simulink model "t2_5_1"  (R2017b)
settings: Solver=VariableStepAuto  StartTime=0.0  StopTime=10.0  RelTol=1e-3
settings Model: Creator=zxy19  LastModifiedBy=zxy19

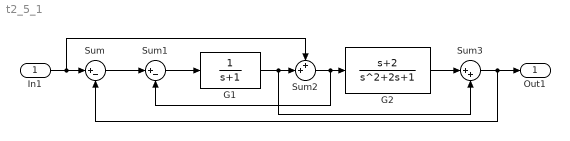
== system t2_5_1 ==
  In1 : Inport
  G1 : TransferFcn  Denominator=[1 1]  ContinuousStateAttributes='G1'
  G2 : TransferFcn  Numerator=[1 2]
  Sum : Sum  Inputs=|+-
  Sum1 : Sum  Inputs=|+-
  Sum2 : Sum  Inputs=++|
  Sum3 : Sum  Inputs=|++
  Out1 : Outport
  wires:
  Sum2/1 -> Sum1/2, G2/1
  G2/1 -> Sum3/1
  Sum3/1 -> Sum/2, Out1/1
  G1/1 -> Sum3/2, Sum2/2
  In1/1 -> Sum2/1, Sum/1
  Sum/1 -> Sum1/1
  Sum1/1 -> G1/1
